simulink model "SigmaDeltaObserverTest"  (R2017a)
settings: Solver=VariableStepAuto  StartTime=0.0  StopTime=100  RelTol=1e-3
settings Model: Creator=bhannigan  LastModifiedBy=bhannigan

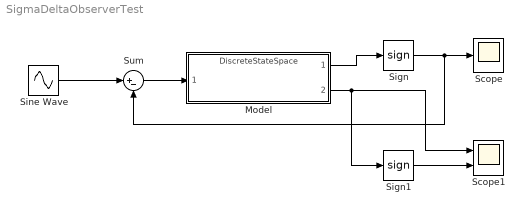
== system SigmaDeltaObserverTest ==
  Model : ModelReference  ModelNameDialog=DiscreteStateSpace  SimulationMode=Normal  ModelReferenceVersion=1.12
  Scope : Scope
  Scope1 : Scope  NumInputPorts=2
  Sign : Signum
  Sign1 : Signum
  Sine Wave : Sin  Frequency=0.1  SampleTime=0
  Sum : Sum  Inputs=|+-
  wires:
  Sine Wave/1 -> Sum/1
  Sum/1 -> Model/1
  Model/1 -> Sign/1
  Model/2 -> Sign1/1, Scope1/1
  Sign/1 -> Scope/1, Sum/2
  Sign1/1 -> Scope1/2
